simulink library "Pressure_Drop_staticHeight"  (R2018b)
settings: Solver=ode45  StartTime=0.0  StopTime=10.0  RelTol=1e-3  EnableMultiTasking=on
undefined symbols (not defined in the file): DPConstant, DPLinear, DPQuadratic, GeodeticHeight, Pressure
libraries: carnot x2, simulink x1
settings Model: Creator=lena.frank  LastModifiedBy=P41573
settings DataIOCC: LimitDataPoints=on  SaveFormat=Array  SignalLoggingSaveFormat=ModelDataLogs
settings OptimizationCC: ExpressionDepthLimit=2147483647  LifeSpan=inf
settings DebuggingCC: UnderspecifiedInitializationDetection=Classic  MergeDetectMultiDrivingBlocksExec=none  SolverPrmCheckMsg=warning  FcnCallInpInsideContextMsg=warning  StateNameClashWarn=warning  SFUnexpectedBacktrackingDiag=warning  SFNoUnconditionalDefaultTransitionDiag=warning  SFExecutionAtInitializationDiag=none
settings HardwareCC: ProdBitPerPointer=32  ProdBitPerSizeT=32  ProdBitPerPtrDiffT=32  ProdLargestAtomicFloat=None  ProdIntDivRoundTo=Undefined  ProdEndianess=Unspecified  ProdWordSize=32  ProdHWDeviceType=32-bit Generic
settings ModelReferenceCC: PropagateSignalLabelsOutOfModel=off
settings SFSimCC: SimUseLocalCustomCode=off
settings RTWCC: RTWUseLocalCustomCode=off
settings CodeAppCC: StateflowObjectComments=on
settings GRTTargetCC: TargetLangStandard=C89/C90 (ANSI)  GeneratePreprocessorConditionals=Disable all  CombineOutputUpdateFcns=off  GRTInterface=on
settings ConfigComp: CovMetricSettings=dw  CovHtmlReporting=on  CovSaveCumulativeToWorkspaceVar=on  CovSaveSingleToWorkspaceVar=on  CovExternalEMLEnable=off

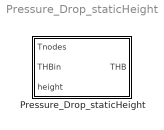
== system Pressure_Drop_staticHeight ==
  Pressure_Drop_staticHeight : Subsystem  mask(Pressure Drop static Height){}
      mask help:
      | Pressure drop or increase due to statig height.
      | Calculation is done for ID > 20000 (dp = f(h)).
      | dp = height/Nnodes*grav*density(Tnodes)
      | The length of Tnodes defines the number of temperature nodes.
      | The height is between inlet and outlet. It is divided by the number of nodes Nnodes in the temperature vector "Tnodes".
      | Height is positive for outlet above inlet when pressure decreases.
      mask Help: web(fullfile(path_carnot('help'),'Pressure_Drop_staticHeight.html'),'-helpbrowser')

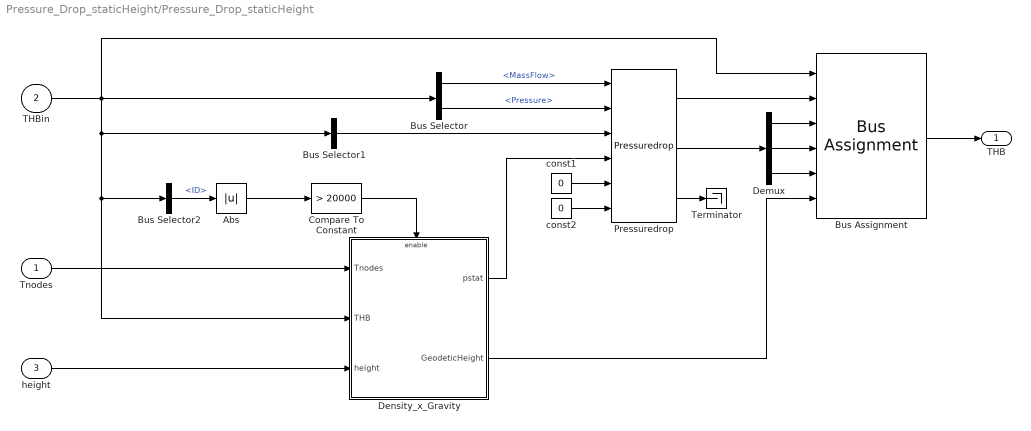
== system Pressure_Drop_staticHeight/Pressure_Drop_staticHeight ==
  Tnodes : Inport
  THBin : Inport  Port=2
  height : Inport  Port=3
  Abs : Abs
  Bus Assignment : BusAssignment  AssignedSignals=Pressure,DPConstant,DPLinear,DPQuadratic,GeodeticHeight
  Bus Selector : BusSelector  OutputSignals=MassFlow,Pressure
  Bus Selector1 : BusSelector  OutputSignals=DPConstant,DPLinear,DPQuadratic  OutputAsBus=on
  Bus Selector2 : BusSelector  OutputSignals=ID
  Compare To Constant : simulink/Logic and Bit Operations/Compare To Constant  relop=>  const=20000  OutDataTypeStr=boolean
  Demux : Demux  Outputs=3
  Density_x_Gravity : Subsystem
  Pressuredrop : carnot/Basic/Pressure_Drop/Pressuredrop
      settings: SourceProductName=Carnot
  Terminator : Terminator
  const1 : Constant  Value=0
  const2 : Constant  Value=0
  THB : Outport
  wires:
  const2/1 -> Pressuredrop/6
  const1/1 -> Pressuredrop/5
  Pressuredrop/3 -> Terminator/1
  Density_x_Gravity/1(pstat) -> Pressuredrop/4
  Compare To Constant/1 -> Density_x_Gravity/Enable
  Tnodes/1 -> Density_x_Gravity/1(Tnodes)
  Bus Selector2/1 -> Abs/1  "<ID>"
  Bus Selector/2 -> Pressuredrop/2  "<Pressure>"
  Bus Selector/1 -> Pressuredrop/1  "<MassFlow>"
  Bus Selector1/1 -> Pressuredrop/3
  Abs/1 -> Compare To Constant/1
  THBin/1 -> Bus Selector2/1, Density_x_Gravity/2(THB), Bus Selector1/1, Bus Selector/1, Bus Assignment/1
  Bus Assignment/1 -> THB/1
  Pressuredrop/1 -> Bus Assignment/2
  Demux/1 -> Bus Assignment/3
  Demux/2 -> Bus Assignment/4
  Demux/3 -> Bus Assignment/5
  Pressuredrop/2 -> Demux/1
  height/1 -> Density_x_Gravity/3(height)
  Density_x_Gravity/2(GeodeticHeight) -> Bus Assignment/6

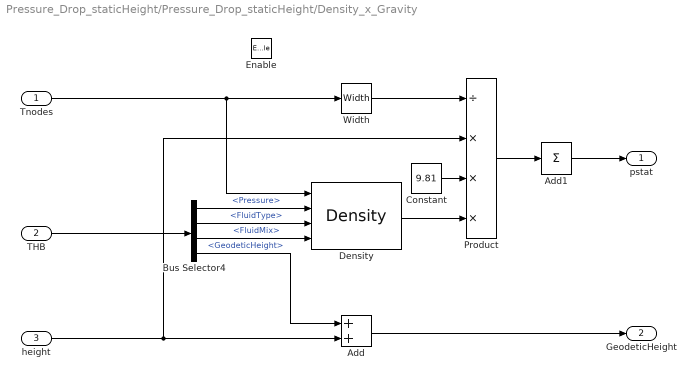
== system Pressure_Drop_staticHeight/Pressure_Drop_staticHeight/Density_x_Gravity ==
  Tnodes : Inport
  THB : Inport  Port=2
  height : Inport  Port=3
  Enable : EnablePort
  Add : Sum
  Add1 : Sum  Inputs=1
  Bus Selector4 : BusSelector  OutputSignals=Pressure,FluidType,FluidMix,GeodeticHeight
  Constant : Constant  Value=9.81
  Density : carnot/Basic/Material_Properties/Density  VariantControl=CarlibClassic  INPUTARGUMENTS=state variables (classic)  DEBUGLEVEL=DEBUGLEVEL  MAXTOTALWARNINGS=inf  MAXCONSECUTIVEWARNINGS=inf  WRITETOFILE=0  FILENAME='errors.txt'
      settings: SourceProductName=Carnot
  Product : Product  Inputs=/***  RndMeth=Zero
  Width : Width
  pstat : Outport
  GeodeticHeight : Outport  Port=2
  wires:
  Bus Selector4/1 -> Density/2  "<Pressure>"
  Bus Selector4/2 -> Density/3  "<FluidType>"
  Bus Selector4/3 -> Density/4  "<FluidMix>"
  THB/1 -> Bus Selector4/1
  Tnodes/1 -> Density/1, Width/1
  Bus Selector4/4 -> Add/1  "<GeodeticHeight>"
  height/1 -> Add/2, Product/2
  Add/1 -> GeodeticHeight/1
  Width/1 -> Product/1
  Density/1 -> Product/4
  Product/1 -> Add1/1
  Constant/1 -> Product/3
  Add1/1 -> pstat/1
